simulink model "Simulink_03_10"  (R2024a)
settings: Solver=VariableStepAuto  StartTime=0.0  StopTime=2.5  RelTol=1e-3
undefined symbols (not defined in the file): km, kp, tau, Td, Theta10, Theta20, Ti
libraries: slpidlib x1
settings Model: Creator=cocoma-reyes  LastModifiedBy=cocoma-reyes

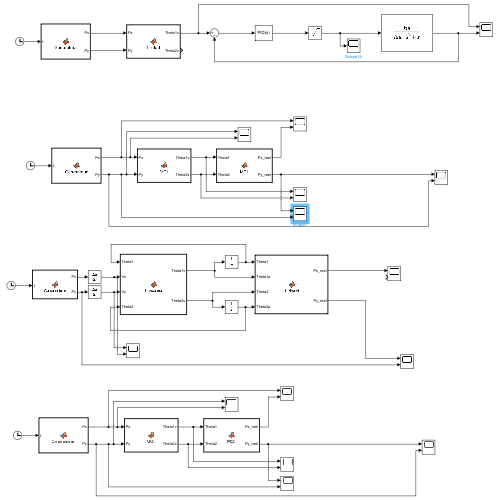
[thumbnail: Simulink's stored preview of the top-level diagram]
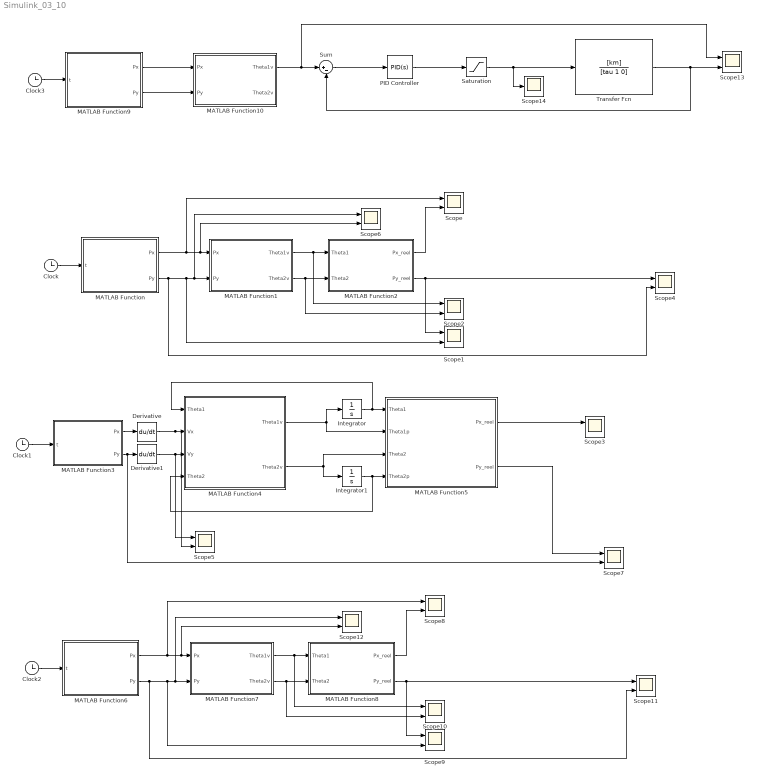
== system Simulink_03_10 ==
  Clock{,1..3} (4 alike) : Clock
  Derivative : Derivative
  Derivative1 : Derivative
  Integrator : Integrator  InitialCondition=Theta10
  Integrator1 : Integrator  InitialCondition=Theta20
  MATLAB Function : MATLAB Function  TreatAsAtomicUnit=on
  MATLAB Function1 : MATLAB Function  TreatAsAtomicUnit=on
  MATLAB Function10 : MATLAB Function  TreatAsAtomicUnit=on
  MATLAB Function2 : MATLAB Function  TreatAsAtomicUnit=on
  MATLAB Function3 : MATLAB Function  TreatAsAtomicUnit=on
  MATLAB Function4 : MATLAB Function  TreatAsAtomicUnit=on
  MATLAB Function5 : MATLAB Function  TreatAsAtomicUnit=on
  MATLAB Function6 : MATLAB Function  TreatAsAtomicUnit=on
  MATLAB Function7 : MATLAB Function  TreatAsAtomicUnit=on
  MATLAB Function8 : MATLAB Function  TreatAsAtomicUnit=on
  MATLAB Function9 : MATLAB Function  TreatAsAtomicUnit=on
  PID Controller : slpidlib/PID Controller  Controller=PID  Form=Parallel  TimeDomain=Continuous-time  UseExternalTs=off  SampleTime=-1  IntegratorMethod=Forward Euler  FilterMethod=Forward Euler  ControllerParametersSource=internal  P=kp  I=Ti  UseKiTs=off  D=Td  UseExternalDerivativeSource=off  N=100  UseFilter=on  TunerSelectOption=Transfer Function Based (PID Tuner App)  InitialConditionSource=internal  InitialConditionForIntegrator=0  InitialConditionForFilter=0  DifferentiatorICPrevScaledInput=0  ExternalReset=none  TrackingMode=off  Kt=1  LimitOutput=off  SatLimitsSource=internal  UpperSaturationLimit=inf  LowerSaturationLimit=-inf  LinearizeAsGain=on  AntiWindupMode=none  Kb=1  LimitIntegrator=off  UpperIntegratorSaturationLimit=inf  LowerIntegratorSaturationLimit=-inf  POutMin=[]  POutMax=[]  IOutMin=[]  IOutMax=[]  DOutMin=[]  DOutMax=[]  NOutMin=[]  NOutMax=[]  SumOutMin=[]  SumOutMax=[]  SaturationOutMin=[]  SaturationOutMax=[]  PParamMin=[]  PParamMax=[]  IParamMin=[]  IParamMax=[]  DParamMin=[]  DParamMax=[]  NParamMin=[]  NParamMax=[]  KbParamMin=[]  KbParamMax=[]  KtParamMin=[]  KtParamMax=[]  KbOutMin=[]  KbOutMax=[]  KtOutMin=[]  KtOutMax=[]  IntegratorOutMin=[]  IntegratorOutMax=[]  FilterOutMin=[]  FilterOutMax=[]  SumI1OutMin=[]  SumI1OutMax=[]  SumI2OutMin=[]  SumI2OutMax=[]  SumI3OutMin=[]  SumI3OutMax=[]  SumI4OutMin=[]  SumI4OutMax=[]  SumDOutMin=[]  SumDOutMax=[]  DifferentiatorOutMin=[]  DifferentiatorOutMax=[]  FilterDiffOutCoefMin=[]  FilterDiffOutCoefMax=[]  ReciprocalOutMin=[]  ReciprocalOutMax=[]  SumDenOutMin=[]  SumDenOutMax=[]  SumNumOutMin=[]  SumNumOutMax=[]  DivideOutMin=[]  DivideOutMax=[]  UdiffTsProdOutMin=[]  UdiffTsProdOutMax=[]  NTsProdOutMin=[]  NTsProdOutMax=[]  UintegralTsProdOutMin=[]  UintegralTsProdOutMax=[]  UngainTsProdOutMin=[]  UngainTsProdOutMax=[]  ClampingZeroOutDataTypeStr=Inherit: Inherit via back propagation  ClampingZeroOutMin=[]  ClampingZeroOutMax=[]  FilterDenConstantOutDataTypeStr=Inherit: Inherit via back propagation  FilterDenConstantOutMin=[]  FilterDenConstantOutMax=[]  PCopyOutDataTypeStr=Inherit: Inherit via back propagation  PCopyOutMin=[]  PCopyOutMax=[]  NCopyOutDataTypeStr=Inherit: Inherit via back propagation  NCopyOutMin=[]  NCopyOutMax=[]  IntegratorContinuousStateAttributes=''  IntegratorStateMustResolveToSignalObject=off  IntegratorRTWStateStorageClass=Auto  FilterContinuousStateAttributes=''  FilterStateMustResolveToSignalObject=off  FilterRTWStateStorageClass=Auto  ParallelPVariant=InternalParameters  IdealPVariant=Disabled  IVariant=InternalParameters  DVariant=InternalParameters  IntegratorVariant=Continuous  SatVariant=Disabled  AWVariant=Passthrough  PCopyVariant=Disabled  TRVariant=Disabled  FdbkBlocksVariant=Forward  IdealPFdbkVariant=Disabled  SatFdbkVariant=Disabled  DerivativeFilterVariant=ContFilter  NVariant=InternalParameters  NCopyVariant=Disabled  FilterICVariant=InternalICsFilter  IntegratorICVariant=InternalICs  ExternalResetVariant=Disabled  TRSumVariant=Passthrough  SumFdbkVariant=Disabled  SumVariant=Sum_PID  TsampFilterVariant=InternalTs  TsampNgainVariant=Passthrough  TsampIntegralVariant=Disabled_SignalSpec  ExternalSaturationOutDataTypeStr=Inherit: Same as second input  DerivativeSourceVariant=ErrorSignal
  Saturation : Saturate  UpperLimit=10  LowerLimit=-10
  Scope{,1..13} (14 alike) : Scope  NumInputPorts=2
  Scope14 : Scope
  Sum : Sum  Inputs=|+-
  Transfer Fcn : TransferFcn  Numerator=[km]  Denominator=[tau 1 0]
  wires:
  MATLAB Function1/1(Theta1v) -> Scope2/1, MATLAB Function2/1(Theta1)
  MATLAB Function1/2(Theta2v) -> Scope2/2, MATLAB Function2/2(Theta2)
  Clock/1 -> MATLAB Function/1(t)
  MATLAB Function/1(Px) -> Scope/1, Scope6/2, MATLAB Function1/1(Px)
  MATLAB Function2/2(Py_reel) -> Scope4/1, Scope1/1
  MATLAB Function2/1(Px_reel) -> Scope/2
  MATLAB Function5/1(Px_reel) -> Scope3/1
  MATLAB Function4/2(Theta2v) -> MATLAB Function5/3(Theta2), Integrator1/1
  Clock1/1 -> MATLAB Function3/1(t)
  MATLAB Function4/1(Theta1v) -> MATLAB Function5/2(Theta1p), Integrator/1
  MATLAB Function5/2(Py_reel) -> Scope7/1
  Integrator/1 -> MATLAB Function4/1(Theta1), MATLAB Function5/1(Theta1)
  Integrator1/1 -> MATLAB Function5/4(Theta2p), MATLAB Function4/4(Theta2)
  MATLAB Function3/1(Px) -> Derivative/1
  MATLAB Function3/2(Py) -> Scope7/2, Derivative1/1
  Derivative/1 -> Scope5/2, MATLAB Function4/2(Vx)
  Derivative1/1 -> Scope5/1, MATLAB Function4/3(Vy)
  MATLAB Function/2(Py) -> Scope4/2, Scope1/2, Scope6/1, MATLAB Function1/2(Py)
  MATLAB Function7/1(Theta1v) -> Scope10/1, MATLAB Function8/1(Theta1)
  MATLAB Function6/2(Py) -> Scope11/2, Scope9/2, Scope12/1, MATLAB Function7/2(Py)
  MATLAB Function7/2(Theta2v) -> Scope10/2, MATLAB Function8/2(Theta2)
  MATLAB Function6/1(Px) -> Scope8/1, Scope12/2, MATLAB Function7/1(Px)
  MATLAB Function8/2(Py_reel) -> Scope11/1, Scope9/1
  MATLAB Function8/1(Px_reel) -> Scope8/2
  Clock2/1 -> MATLAB Function6/1(t)
  MATLAB Function9/1(Px) -> MATLAB Function10/1(Px)
  MATLAB Function9/2(Py) -> MATLAB Function10/2(Py)
  Clock3/1 -> MATLAB Function9/1(t)
  Sum/1 -> PID Controller/1
  MATLAB Function10/1(Theta1v) -> Scope13/1, Sum/1
  Saturation/1 -> Scope14/1, Transfer Fcn/1
  Transfer Fcn/1 -> Sum/2, Scope13/2
  PID Controller/1 -> Saturation/1

== matlab function Simulink_03_10/MATLAB Function9 ==
  data: t input; Px output; Py output
function [Px , Py] = Generateur(t)
    V = 0.5;
    A = 2;
    y0 = -0.5;
    y1 = +0.5;
    tau = V/A;
    T = (y1 - y0)/V - tau;
    if t <= tau
        Py = (1/2) * A * t^2 + y0;
    elseif t >= tau && t <= tau + T
        Py = V * (t - tau/2) + y0;
    elseif t >= T + tau && t <= T + 2*tau
        Py = -(1/2) * A * (t - 2*tau - T)^2 + y1;
    else
        Py=y1;
    end
    
    Px = 0.3;
end

== matlab function Simulink_03_10/MATLAB Function1 ==
  data: Px input; Theta1v output; Py input; Theta2v output
function [Theta1v, Theta2v] = MGI(Px,Py)
l1 = 0.3;
l2 = 0.3;

Theta2v = acos((Px^2 + Py^2 - l1^2 - l2^2)/(2*l1*l2));
Theta1v = atan2(-l2*sin(Theta2v)*Px + (l1+l2*cos(Theta2v))*Py,l2*sin(Theta2v)*Py + (l1 + l2*cos(Theta2v))*Px);
end

== matlab function Simulink_03_10/MATLAB Function ==
  data: t input; Px output; Py output
function [Px , Py] = Generateur(t)
    V = 0.5;
    A = 2;
    y0 = -0.5;
    y1 = +0.5;
    tau = V/A;
    T = (y1 - y0)/V - tau;
    if t <= tau
        Py = (1/2) * A * t^2 + y0;
    elseif t >= tau && t <= tau + T
        Py = V * (t - tau/2) + y0;
    elseif t >= T + tau && t <= T + 2*tau
        Py = -(1/2) * A * (t - 2*tau - T)^2 + y1;
    else
        Py=y1;
    end
    
    Px = 0.3;
end

== matlab function Simulink_03_10/MATLAB Function2 ==
  data: Theta1 input; Px_reel output; Theta2 input; Py_reel output
function [Px_reel,Py_reel] = MGI(Theta1,Theta2)
l1 = 0.3;
l2 = 0.3;
Px_reel = l1 * cos(Theta1) + l2 * cos(Theta1 + Theta2);
Py_reel = l1 * sin(Theta1) + l2 * sin(Theta1 + Theta2);
end

== matlab function Simulink_03_10/MATLAB Function3 ==
  data: t input; Px output; Py output
function [Px , Py] = Generateur(t)
    V = 0.5;
    A = 2;
    y0 = -0.5;
    y1 = +0.5;
    tau = V/A;
    T = (y1 - y0)/V - tau;
    if t <= tau
        Py = (1/2) * A * t^2 + y0;
    elseif t >= tau && t <= tau + T
        Py = V * (t - tau/2) + y0;
    elseif t >= T + tau && t <= T + 2*tau
        Py = -(1/2) * A * (t - 2*tau - T)^2 + y1;
    else
        Py=y1;
    end
    
    Px = 0.3;
end

== matlab function Simulink_03_10/MATLAB Function4 ==
  data: Theta1 input; Vx input; Theta1v output; Vy input; Theta2v output; Theta2 input
function [Theta1v, Theta2v] = J_inverse(Theta1, Vx,Vy, Theta2)
l1 = 0.3;
l2 = 0.3;
det = l1 *l2*sin(Theta2);
Theta1v = Vx * ((l2*cos(Theta1+Theta2) - l1*cos(Theta1) + l2*cos(Theta1+Theta2))/det);
Theta2v = Vy * ((l2*sin(Theta1+Theta2) - l1*sin(Theta1) - l2*sin(Theta1+Theta2))/det);
end

== matlab function Simulink_03_10/MATLAB Function5 ==
  data: Theta1 input; Theta1p input; Theta2 input; Theta2p input; Px_reel output; Py_reel output
function [Px_reel, Py_reel] = J_direct(Theta1, Theta1p, Theta2, Theta2p)
l1 = 0.3;
l2 = 0.3;

% Calcul de la position du point final (cinématique directe)
Px_reel = -sin(Theta1)*((l1 +l2)*Theta1p + l2 * Theta2p);
Py_reel = cos(Theta1) * ((l1+l2)*Theta1p + l2 * Theta2p);
end

== matlab function Simulink_03_10/MATLAB Function6 ==
  data: t input; Px output; Py output
function [Px , Py] = Generateur(t)
    V = 0.5;
    A = 2;
    y0 = -0.5;
    y1 = +0.5;
    tau = V/A;
    T = (y1 - y0)/V - tau;
    if t <= tau
        Py = (1/2) * A * t^2 + y0;
    elseif t >= tau && t <= tau + T
        Py = V * (t - tau/2) + y0;
    elseif t >= T + tau && t <= T + 2*tau
        Py = -(1/2) * A * (t - 2*tau - T)^2 + y1;
    else
        Py=y1;
    end
    
    Px = 0.3;
end

== matlab function Simulink_03_10/MATLAB Function7 ==
  data: Px input; Theta1v output; Py input; Theta2v output
function [Theta1v, Theta2v] = MGI(Px,Py)
l1 = 0.3;
l2 = 0.3;

Theta2v = acos((Px^2 + Py^2 - l1^2 - l2^2)/(2*l1*l2));
Theta1v = atan2(-l2*sin(Theta2v)*Px + (l1+l2*cos(Theta2v))*Py,l2*sin(Theta2v)*Py + (l1 + l2*cos(Theta2v))*Px);
end

== matlab function Simulink_03_10/MATLAB Function8 ==
  data: Theta1 input; Px_reel output; Theta2 input; Py_reel output
function [Px_reel,Py_reel] = MGI(Theta1,Theta2)
l1 = 0.3;
l2 = 0.3;
Px_reel = l1 * cos(Theta1) + l2 * cos(Theta1 + Theta2);
Py_reel = l1 * sin(Theta1) + l2 * sin(Theta1 + Theta2);
end

== matlab function Simulink_03_10/MATLAB Function10 ==
  data: Px input; Theta1v output; Py input; Theta2v output
function [Theta1v, Theta2v] = Thetad(Px,Py)
l1 = 0.3;
l2 = 0.3;

Theta2v = acos((Px^2 + Py^2 - l1^2 - l2^2)/(2*l1*l2));
Theta1v = atan2(-l2*sin(Theta2v)*Px + (l1+l2*cos(Theta2v))*Py,l2*sin(Theta2v)*Py + (l1 + l2*cos(Theta2v))*Px);
end
